simulink model "tempModel_agg_heatSource2"  (Simulink 10.0)
settings: Solver=FixedStepAuto  StartTime=0.0  StopTime=3600  FixedStep=fixedStep  MaxStep=0.2  RelTol=1e-3
values from neighbouring files (symbols this model uses):
  parameters1 = [coffeeDiffTemp,0,lambda]    [coffeeMakerInit.m]
  parameters2 = [ovenDiffTemp,0,lambda]    [ovenInit.m]
  parameters3 = [dryerDiffTemp,0,lambda]    [dryerInit.m]
  x01 = t0    [coffeeMakerInit.m]
  x02 = t0    [ovenInit.m]
  x03 = t0    [dryerInit.m]
  xPC = t0    [pressureCookerInit.m]
undefined symbols (not defined in the file or in its folder): lambda, pCookerDiffTemp, startCoffee, startDryer, startOven, startPCooker, timeCoffee, timeDryer, timeOven, timePCooker, xx
settings Model: Creator=lixuansong  LastModifiedBy=lixuansong
settings DataIOCC: SaveFormat=Dataset  ReturnWorkspaceOutputs=on
settings OptimizationCC: LifeSpan=auto
settings DebuggingCC: UnderspecifiedInitializationDetection=Simplified  MergeDetectMultiDrivingBlocksExec=error  SFUnexpectedBacktrackingDiag=error  SFNoUnconditionalDefaultTransitionDiag=error  SFExecutionAtInitializationDiag=warning  ArithmeticOperatorsInVariantConditions=error
settings HardwareCC: ProdBitPerPointer=64  ProdBitPerSizeT=64  ProdBitPerPtrDiffT=64  ProdLargestAtomicFloat=Float  ProdIntDivRoundTo=Zero  ProdEndianess=LittleEndian  ProdWordSize=64  ProdHWDeviceType=Intel->x86-64 (Windows64)
settings ModelReferenceCC: PropagateSignalLabelsOutOfModel=on
settings SFSimCC: SimUseLocalCustomCode=on  CustomCodeUndefinedFunction=FilterOut
settings RTWCC: RTWUseLocalCustomCode=on
settings CodeAppCC: StateflowObjectComments=off
settings GRTTargetCC: TargetLangStandard=C99 (ISO)  CombineOutputUpdateFcns=on  GRTInterface=off
settings ConfigComp: CovMetricSettings=dwe  CovHtmlReporting=off  CovSaveCumulativeToWorkspaceVar=off  CovSaveSingleToWorkspaceVar=off

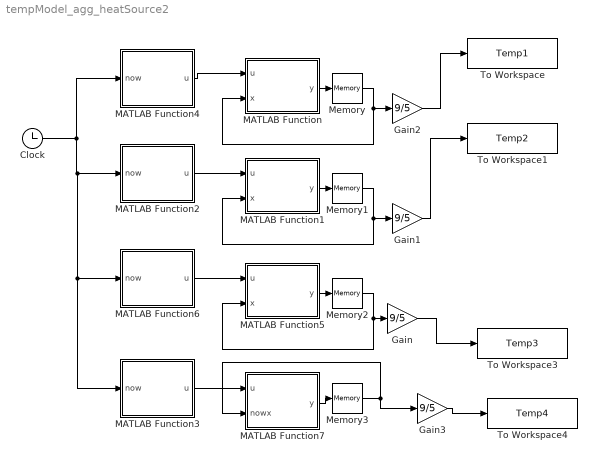
== system tempModel_agg_heatSource2 ==
  Clock : Clock
  Gain{,1..3} (4 alike) : Gain  Gain=9/5
  MATLAB Function : MATLAB Function  TreatAsAtomicUnit=on
  MATLAB Function1 : MATLAB Function  TreatAsAtomicUnit=on
  MATLAB Function2 : MATLAB Function  TreatAsAtomicUnit=on
  MATLAB Function3 : MATLAB Function  TreatAsAtomicUnit=on
  MATLAB Function4 : MATLAB Function  TreatAsAtomicUnit=on
  MATLAB Function5 : MATLAB Function  TreatAsAtomicUnit=on
  MATLAB Function6 : MATLAB Function  TreatAsAtomicUnit=on
  MATLAB Function7 : MATLAB Function  TreatAsAtomicUnit=on
  Memory : Memory  InitialCondition=x01
  Memory1 : Memory  InitialCondition=x02
  Memory2 : Memory  InitialCondition=x03
  Memory3 : Memory  InitialCondition=xPC
  To Workspace : ToWorkspace  VariableName=Temp1  SampleTime=-1
  To Workspace1 : ToWorkspace  VariableName=Temp2  SampleTime=-1
  To Workspace3 : ToWorkspace  VariableName=Temp3  SampleTime=-1
  To Workspace4 : ToWorkspace  VariableName=Temp4  SampleTime=-1
  wires:
  MATLAB Function/1(y) -> Memory/1
  Memory/1 -> MATLAB Function/2(x), Gain2/1
  MATLAB Function4/1(u) -> MATLAB Function/1(u)
  Clock/1 -> MATLAB Function4/1(now), MATLAB Function3/1(now), MATLAB Function6/1(now), MATLAB Function2/1(now)
  MATLAB Function1/1(y) -> Memory1/1
  Memory1/1 -> Gain1/1, MATLAB Function1/2(x)
  MATLAB Function2/1(u) -> MATLAB Function1/1(u)
  MATLAB Function6/1(u) -> MATLAB Function5/1(u)
  Memory2/1 -> Gain/1, MATLAB Function5/2(x)
  MATLAB Function5/1(y) -> Memory2/1
  Gain2/1 -> To Workspace/1
  Gain1/1 -> To Workspace1/1
  Gain/1 -> To Workspace3/1
  Memory3/1 -> MATLAB Function7/2(nowx), Gain3/1
  Gain3/1 -> To Workspace4/1
  MATLAB Function7/1(y) -> Memory3/1
  MATLAB Function3/1(u) -> MATLAB Function7/1(u)

== matlab function MATLAB Function1 ==
  data: u input double; y output double; x input double; parameters2 parameter double; xx parameter double
function y = oven(u,x,parameters2, xx)




tL=parameters2(:,1);
tR=parameters2(:,2);
lambda=parameters2(:,3);


    temp1=x;
    
        
    
             for i = 1:length(xx) % for space steps
                if i == 1
                    temp1(i) = u*tL;
              %     temp1(i) = tL;
                elseif i == length(xx)
                    temp1(i) = tR;
                else 
                    temp1(i) = temp1(i)+lambda*(temp1(i+1)-2*temp1(i)+temp1(i-1));
                end
            end
y = temp1;

== matlab function MATLAB Function ==
  data: u input double; y output double; x input double; parameters1 parameter double; xx parameter double
function y = coffeeMaker(u,x,parameters1, xx)




tL=parameters1(:,1);
tR=parameters1(:,2);
lambda=parameters1(:,3);


    temp1=x;
    
        
    
             for i = 1:length(xx) % for space steps
                if i == 1
                    temp1(i) = u*tL;
              %     temp1(i) = tL;
                elseif i == length(xx)
                    temp1(i) = tR;
                else 
                    temp1(i) = temp1(i)+lambda*(temp1(i+1)-2*temp1(i)+temp1(i-1));
                end
            end
y = temp1;

== matlab function MATLAB Function2 ==
  data: u output double; now input double; startOven parameter double; timeOven parameter double
function u = controlOven(now,startOven, timeOven)
if now>=startOven && now<=startOven+timeOven
    u=1;
else
    u=0;
end

== matlab function MATLAB Function4 ==
  data: u output double; now input double; startCoffee parameter double; timeCoffee parameter double
function u = controlCoffee(now,startCoffee,timeCoffee)
if now>=startCoffee && now<=startCoffee+timeCoffee
    u=1;
else
    u=0;
end

== matlab function MATLAB Function5 ==
  data: u input double; y output double; x input double; parameters3 parameter double; xx parameter double
function y = dryer(u,x,parameters3, xx)




tL=parameters3(:,1);
tR=parameters3(:,2);
lambda=parameters3(:,3);


    temp1=x;
    
        
    
             for i = 1:length(xx) % for space steps
                if i == 1
                    temp1(i) = u*tL;
              %     temp1(i) = tL;
                elseif i == length(xx)
                    temp1(i) = tR;
                else 
                    temp1(i) = temp1(i)+lambda*(temp1(i+1)-2*temp1(i)+temp1(i-1));
                end
            end
y = temp1;

== matlab function MATLAB Function6 ==
  data: u output double; now input double; startDryer parameter double; timeDryer parameter double
function u = controlDryer(now,startDryer, timeDryer)
if now>=startDryer && now<=startDryer+timeDryer
    u=1;
else
    u=0;
end

== matlab function MATLAB Function3 ==
  data: u output double; now input double; startPCooker parameter double; timePCooker parameter double
function u = controlDevice(now,startPCooker,timePCooker)


if now>=startPCooker && now<=startPCooker+timePCooker
    u=1;
else
    u=0;
end

== matlab function MATLAB Function7 ==
  data: u input double; y output double; nowx input double; pCookerDiffTemp parameter double; xx parameter double; lambda parameter double
function y = deviceExe(u,nowx,pCookerDiffTemp, xx, lambda)





    temp1=nowx;
    
        
    
             for i = 1:length(xx) % for space steps
                if i == 1
                    temp1(i) = u*pCookerDiffTemp;
              %     temp1(i) = tL;
                elseif i == length(xx)
                    temp1(i) = 0;
                else 
                    temp1(i) = temp1(i)+lambda*(temp1(i+1)-2*temp1(i)+temp1(i-1));
                end
             end
    y = temp1;
end
